simulink model "AdditionalPump_series"  (R2016b)
settings: Solver=ode45  StartTime=0.0  StopTime=200  MaxStep=5  RelTol=1e-3  EnableMultiTasking=on
undefined symbols (not defined in the file): path_carnot
libraries: carnot x5, simulink x1
settings Model: Creator=drhf  LastModifiedBy=drhf
settings DataIOCC: LimitDataPoints=on  SaveFormat=Array  SignalLoggingSaveFormat=ModelDataLogs
settings OptimizationCC: ExpressionDepthLimit=2147483647  LifeSpan=inf
settings DebuggingCC: UnderspecifiedInitializationDetection=Classic  MergeDetectMultiDrivingBlocksExec=none  SolverPrmCheckMsg=warning  StateNameClashWarn=warning  SFUnexpectedBacktrackingDiag=warning  SFNoUnconditionalDefaultTransitionDiag=warning  SFExecutionAtInitializationDiag=none
settings HardwareCC: ProdBitPerPointer=32  ProdBitPerSizeT=32  ProdBitPerPtrDiffT=32  ProdLargestAtomicFloat=None  ProdIntDivRoundTo=Undefined  ProdEndianess=Unspecified  ProdWordSize=32  ProdHWDeviceType=32-bit Generic
settings ModelReferenceCC: PropagateSignalLabelsOutOfModel=off
settings GRTTargetCC: TargetLangStandard=C89/C90 (ANSI)  GeneratePreprocessorConditionals=Disable all  CombineOutputUpdateFcns=off  GRTInterface=on
settings ConfigComp: CovMetricSettings=dw  CovHtmlReporting=on  CovSaveCumulativeToWorkspaceVar=on  CovSaveSingleToWorkspaceVar=on  CovExternalEMLEnable=off

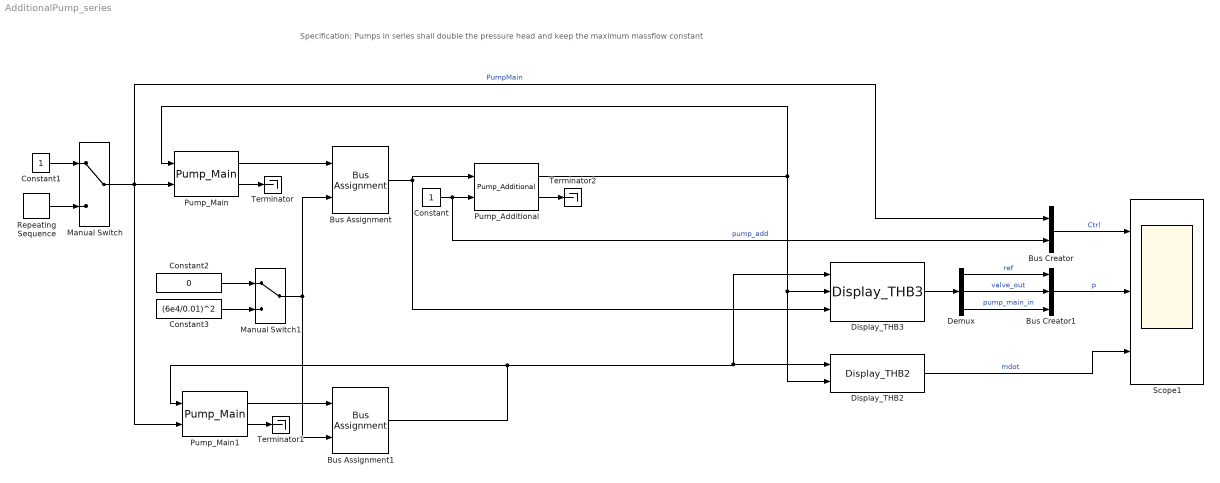
== system AdditionalPump_series ==
  note: Specification:
      | Pumps in series shall double the pressure head and keep the maximum massflow constant
  Bus Assignment : BusAssignment  AssignedSignals=DPQuadratic
  Bus Assignment1 : BusAssignment  AssignedSignals=DPQuadratic
  Bus Creator : BusCreator  Inputs=2
  Bus Creator1 : BusCreator  Inputs=3
  Constant : Constant
  Constant1 : Constant
  Constant2 : Constant  Value=0
  Constant3 : Constant  Value=(6e4/0.01)^2
  Demux : Demux  Outputs=3
  Display_THB2 : carnot/Outputs/Display_THB2  t=off  m=on  p=off  id=off  mix=off  d=off
  Display_THB3 : carnot/Outputs/Display_THB3  t=off  m=off  p=on  id=off  mix=off  d=off
  Manual Switch : ManualSwitch
  Manual Switch1 : ManualSwitch
  Pump_Additional : carnot/Hydraulics/Pump_Additional  Tini=20  PathName=fullfile(path_carnot('libsl'), 'Hydraulics', 'Pump_Main', 'parameter_set')  FileName='Pump6m.mat'  userPath=off  userParam=off  a0=60000  a1=-43200  a2=0  dia=0.025  UA=1  mcp=4182  e0=50  e1=28.8  e2=-10.368
  Pump_Main : carnot/Hydraulics/Pump_Main  Tini=20  p0=3e5  IDpreset=pressure drop  fluid=Water  mix=0  mix2=0  mix3=0  t1=0.1  PathName=fullfile(path_carnot('libsl'), 'Hydraulics', 'Pump_Main', 'parameter_set')  FileName='Pump6m.mat'  userPath=off  userParam=off  a0=60000  a1=-43200  a2=0  dia=0.025  UA=1  mcp=4182  e0=50  e1=28.8  e2=-10.368
  Pump_Main1 : carnot/Hydraulics/Pump_Main  Tini=20  p0=3e5  IDpreset=pressure drop  fluid=Water  mix=0  mix2=0  mix3=0  t1=0.1  PathName=fullfile(path_carnot('libsl'), 'Hydraulics', 'Pump_Main', 'parameter_set')  FileName='Pump6m.mat'  userPath=off  userParam=off  a0=60000  a1=-43200  a2=0  dia=0.025  UA=1  mcp=4182  e0=50  e1=28.8  e2=-10.368
  Repeating Sequence : simulink/Sources/Repeating Sequence  rep_seq_t=[0 20 60 200]  rep_seq_y=[0 0 1 1]
  Scope1 : Scope  NumInputPorts=3
  Terminator : Terminator
  Terminator1 : Terminator
  Terminator2 : Terminator
  wires:
  Pump_Additional/2 -> Terminator2/1
  Manual Switch/1 -> Pump_Main1/2, Bus Creator/1, Pump_Main/2  "PumpMain"
  Pump_Main/2 -> Terminator/1
  Bus Creator/1 -> Scope1/1  "Ctrl"
  Pump_Additional/1 -> Display_THB2/2, Display_THB3/2, Pump_Main/1
  Bus Assignment/1 -> Display_THB3/3, Pump_Additional/1
  Display_THB3/1 -> Demux/1
  Demux/1 -> Bus Creator1/1  "ref"
  Demux/2 -> Bus Creator1/2  "valve_out"
  Demux/3 -> Bus Creator1/3  "pump_main_in"
  Bus Creator1/1 -> Scope1/2  "p"
  Constant/1 -> Bus Creator/2, Pump_Additional/2  "pump_add"
  Repeating Sequence/1 -> Manual Switch/2
  Constant1/1 -> Manual Switch/1
  Pump_Main1/2 -> Terminator1/1
  Bus Assignment1/1 -> Display_THB3/1, Display_THB2/1, Pump_Main1/1
  Manual Switch1/1 -> Bus Assignment/2, Bus Assignment1/2
  Display_THB2/1 -> Scope1/3  "mdot"
  Pump_Main/1 -> Bus Assignment/1
  Pump_Main1/1 -> Bus Assignment1/1
  Constant2/1 -> Manual Switch1/1
  Constant3/1 -> Manual Switch1/2
